simulink model "SolarPanelDigitalTwin_Auto"  (R2025b)
settings: Solver=ode23t  StartTime=0.0  StopTime=6300  MaxStep=4  RelTol=1e-3
libraries: ee_lib x117, fl_lib x9, nesl_utility x7, batteryecm_lib x1
settings Model: Creator=suraj  LastModifiedBy=suraj

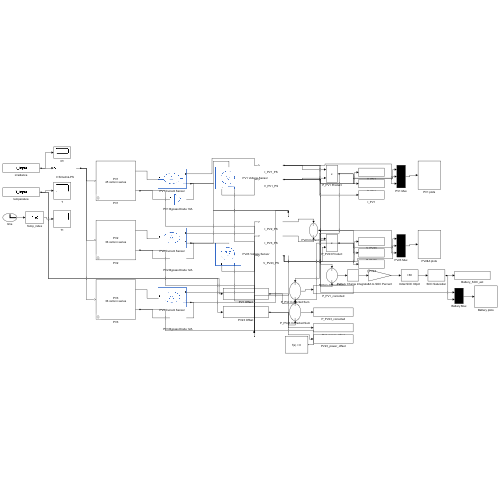
[thumbnail: Simulink's stored preview of the top-level diagram]
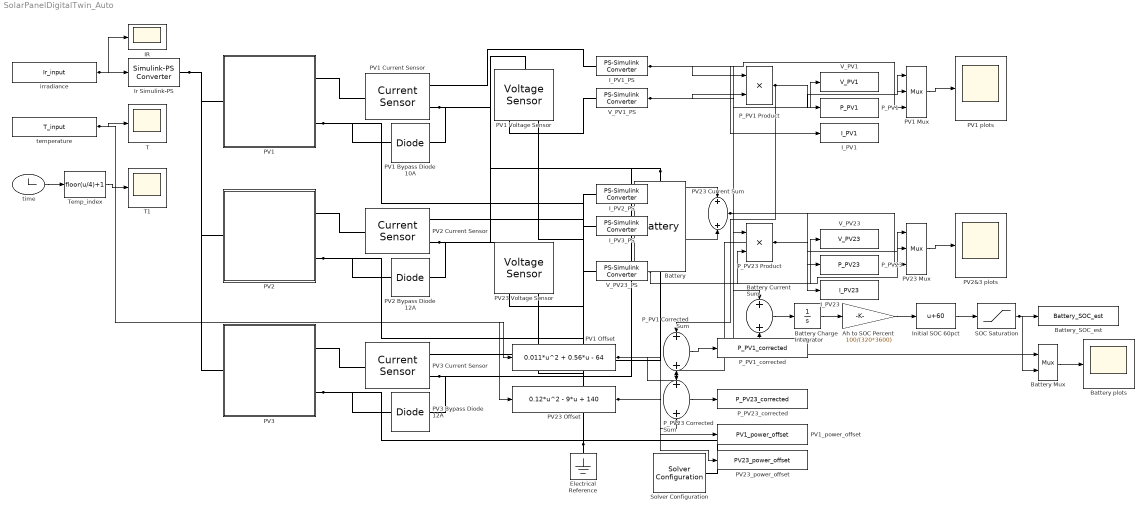
== system SolarPanelDigitalTwin_Auto ==
  Ah to SOC Percent : Gain  Gain=100/(320*3600)
  Battery : batteryecm_lib/Battery  Vnom=12 V  prm_dir=simscape.enum.battery.prm_dir.disabled  R1_dis=2 Ohm  R1_ch=2 Ohm  R1=0.05 Ohm  prm_AH=simscape.enum.battery.prm_AH.infinite  AH=320 A*hr  V1=11.5 V  AH1=25 A*hr  prm_R2=simscape.enum.battery.prm_R2.disabled  R2=2000 Ohm  Tmeas=298.15 K  charge_measurement_port=simscape.enum.battery.enable.no  prm_dyn=simscape.enum.battery.prm_dyn.off  Rp1=0.005 Ohm  tau1=30 s  Rp2=0.005 Ohm  tau2=30 s  Rp3=0.005 Ohm  tau3=30 s  Rp4=0.005 Ohm  tau4=30 s  Rp5=0.005 Ohm  tau5=30 s  prm_fade=simscape.enum.battery.prm_fade.disabled  N_fade=100  AH_fade=45 A*hr  R1_fade=2.02 Ohm  R1_ch_fade=2.02 Ohm  V1_fade=10.35 V  prm_age=simscape.enum.battery.prm_age.disabled  prm_age_OCV=simscape.enum.battery.prm_age_OCV.OCV  OCV_age=0.9  SOC_age=60  Tmeas_age=298.15 K  delta_time_age_vec=[0] d  temperature_age_vec=[273] K  OCV_scaling_age=2.2134e6  OCV_offset_age=1.632e6  temp_exp_age=0.515833569 V  t_exp_age=0.75  Vnom_T2=12 V  R1_T2=2.2 Ohm  R1_T2_dis=2.2 Ohm  R1_T2_ch=2.2 Ohm  V1_T2=11.4 V  R2_T2=2200 Ohm  Rp1_T2=0.005 Ohm  tau1_T2=30 s  Rp2_T2=0.005 Ohm  tau2_T2=30 s  Rp3_T2=0.005 Ohm  tau3_T2=30 s  Rp4_T2=0.005 Ohm  tau4_T2=30 s  Rp5_T2=0.005 Ohm  tau5_T2=30 s  Tmeas2=273.15 K  thermal_port=simscape.enum.thermaleffects.omit  thermal_mass=30000 J/K  i_specify=off  i_priority=None  i=0 A  i_nominal_specify=off  i_nominal_value=1  i_nominal_unit=A  v_specify=off  v_priority=None  v=0 V  v_nominal_specify=off  v_nominal_value=1  v_nominal_unit=V  charge_specify=off  charge_priority=High  charge=50 A*hr  charge_nominal_specify=off  charge_nominal_value=1  charge_nominal_unit=A*hr  num_cycles_specify=off  num_cycles_priority=High  num_cycles=0  num_cycles_nominal_specify=off  num_cycles_nominal_value=1  num_cycles_nominal_unit=1  temperature_specify=off  temperature_priority=High  temperature=298.15 K  temperature_nominal_specify=off  temperature_nominal_value=1  temperature_nominal_unit=K
  Battery Charge Integrator : Integrator
  Battery Current Sum : Sum
  Battery Mux : Mux  Inputs=2
  Battery plots : Scope
  Battery_SOC_est : ToWorkspace  VariableName=Battery_SOC_est  SampleTime=-1
  Electrical Reference : fl_lib/Electrical/Electrical Elements/Electrical Reference
  IR : Scope
  I_PV1 : ToWorkspace  VariableName=I_PV1  SampleTime=-1
  I_PV1_PS : nesl_utility/PS-Simulink Converter  PhysicalDomain=network_engine_domain  SubClassName=ps_output  LeftPortType=input  RightPortType=output  PseudoPeriodic=off  Frequencies=[]  VectorFormat=inherit  Unit=A  AffineConversion=off
  I_PV23 : ToWorkspace  VariableName=I_PV23  SampleTime=-1
  I_PV2_PS : nesl_utility/PS-Simulink Converter  PhysicalDomain=network_engine_domain  SubClassName=ps_output  LeftPortType=input  RightPortType=output  PseudoPeriodic=off  Frequencies=[]  VectorFormat=inherit  Unit=A  AffineConversion=off
  I_PV3_PS : nesl_utility/PS-Simulink Converter  PhysicalDomain=network_engine_domain  SubClassName=ps_output  LeftPortType=input  RightPortType=output  PseudoPeriodic=off  Frequencies=[]  VectorFormat=inherit  Unit=A  AffineConversion=off
  Initial SOC 60pct : Bias  Bias=60  SaturateOnIntegerOverflow=off
  Ir Simulink-PS : nesl_utility/Simulink-PS Converter  PhysicalDomain=network_engine_domain  SubClassName=ps_input  LeftPortType=input  RightPortType=output  PseudoPeriodic=off  Frequencies=[]  NoiseDistribution=none  NoiseParameters=[]  Unit=W/m^2  AffineConversion=off  FilteringAndDerivatives=provide  SimscapeFilterOrder=1  InputFilterTimeConstant=0.001  UdotUserProvided=0
  PV1 : Subsystem  mask{Isc=5.49, Voc=21.5, n=1.5, Rs=0, Ir0=1000, T=40}
      mask prompts: Isc "Short circuit current"; Voc "Open circuit voltage"; n "Quality factor, N"; Rs "Series resistance"; Ir0 "Reference irradiation"; T "Temperature"
      mask Display: disp('PV1\n45 cells in series')
  PV1 Bypass Diode 10A : fl_lib/Electrical/Electrical Elements/Diode  Vf=0.6 V  Ron=0.3 Ohm  Goff=1e-8 1/Ohm  i_specify=off  i_priority=None  i=0 A  i_nominal_specify=off  i_nominal_value=1  i_nominal_unit=A  v_specify=off  v_priority=None  v=0 V  v_nominal_specify=off  v_nominal_value=1  v_nominal_unit=V
  PV1 Current Sensor : fl_lib/Electrical/Electrical Sensors/Current Sensor
  PV1 Mux : Mux  Inputs=3
  PV1 Offset : Fcn  Expr=0.011*u^2 + 0.56*u - 64
  PV1 Voltage Sensor : fl_lib/Electrical/Electrical Sensors/Voltage Sensor
  PV1 plots : Scope
  PV1_power_offset : ToWorkspace  VariableName=PV1_power_offset  SampleTime=-1
  PV2 : Subsystem  mask{Isc=6.37, Voc=21.5, n=1.5, Rs=0, Ir0=1000, T=40}
      mask prompts: Isc "Short circuit current"; Voc "Open circuit voltage"; n "Quality factor, N"; Rs "Series resistance"; Ir0 "Reference irradiation"; T "Temperature"
      mask Display: disp('PV2\n36 cells in series')
  PV2 Bypass Diode 12A : fl_lib/Electrical/Electrical Elements/Diode  Vf=0.6 V  Ron=0.3 Ohm  Goff=1e-8 1/Ohm  i_specify=off  i_priority=None  i=0 A  i_nominal_specify=off  i_nominal_value=1  i_nominal_unit=A  v_specify=off  v_priority=None  v=0 V  v_nominal_specify=off  v_nominal_value=1  v_nominal_unit=V
  PV2 Current Sensor : fl_lib/Electrical/Electrical Sensors/Current Sensor
  PV2&3 plots : Scope
  PV23 Current Sum : Sum
  PV23 Mux : Mux  Inputs=3
  PV23 Offset : Fcn  Expr=0.12*u^2 - 9*u + 140
  PV23 Voltage Sensor : fl_lib/Electrical/Electrical Sensors/Voltage Sensor
  PV23_power_offset : ToWorkspace  VariableName=PV23_power_offset  SampleTime=-1
  PV3 : Subsystem  mask{Isc=6.37, Voc=21.5, n=1.5, Rs=0, Ir0=1000, T=40}
      mask prompts: Isc "Short circuit current"; Voc "Open circuit voltage"; n "Quality factor, N"; Rs "Series resistance"; Ir0 "Reference irradiation"; T "Temperature"
      mask Display: disp('PV3\n36 cells in series')
  PV3 Bypass Diode 12A : fl_lib/Electrical/Electrical Elements/Diode  Vf=0.6 V  Ron=0.3 Ohm  Goff=1e-8 1/Ohm  i_specify=off  i_priority=None  i=0 A  i_nominal_specify=off  i_nominal_value=1  i_nominal_unit=A  v_specify=off  v_priority=None  v=0 V  v_nominal_specify=off  v_nominal_value=1  v_nominal_unit=V
  PV3 Current Sensor : fl_lib/Electrical/Electrical Sensors/Current Sensor
  P_PV1 : ToWorkspace  VariableName=P_PV1  SampleTime=-1
  P_PV1 Corrected Sum : Sum
  P_PV1 Product : Product
  P_PV1_corrected : ToWorkspace  VariableName=P_PV1_corrected  SampleTime=-1
  P_PV23 : ToWorkspace  VariableName=P_PV23  SampleTime=-1
  P_PV23 Corrected Sum : Sum
  P_PV23 Product : Product
  P_PV23_corrected : ToWorkspace  VariableName=P_PV23_corrected  SampleTime=-1
  SOC Saturation : Saturate  UpperLimit=100  LowerLimit=0
  Solver Configuration : nesl_utility/Solver Configuration  PhysicalDomain=network_engine_domain  SubClassName=solver  LeftPortType=input  RightPortType=generic  Tones=[]  Harmonics=[]  SimulateNoise=off  Profile=off  UseLocalSampling=off  EnableSwitchedLinearOptims=on  FrequencyDomain=off  UseCCode=off  RelTol=0.001  AbsTol=0.001  MinStep=1e-09  ToWorkspace=off  RevertToSquareIcSolve=off  NumHomotopyIterations=100  PhasorMode=off  PhasorModeNumHarmonics=1  ConsistencySolver=NEWTON_XTOL_AFTER_FTOL  IndexReductionMethod=DerivativeReplacement  DoDC=on  ResidualTolerance=1e-09  ConsistencyTolSource=GLOBAL  ConsistencyAbsTol=0.001  ConsistencyRelTol=0.001  ConsistencyTolFactor=0.001  UseLocalSolver=off  LocalSolverChoice=NE_BACKWARD_EULER_ADVANCER  ResolveIndetEquations=on  FunctionEvalNumThread=1  LocalSolverSampleTime=4  DoFixedCost=off  MaxNonlinIter=3  MaxModeIter=2  ComputeImpulses=off  ImpulseIterations=2  LinearAlgebra=auto  LinearAlgebraNumThread=0  EquationFormulation=NE_TIME_EF  DelaysMemoryBudget=1024  AutomaticFiltering=on  FilteringTimeConstant=0.001  PartitionStorageMethod=AS_NEEDED  PartitionMemoryBudget=1024  PartitionMethod=ROBUST  MultibodyUseLocalSolver=off  MultibodyLocalSolverChoice=ODE1  MultibodyLocalSolverSampleTime=0.001
  T : Scope
  T1 : Scope
  Temp_index : Fcn  Expr=floor(u/4)+1
  V_PV1 : ToWorkspace  VariableName=V_PV1  SampleTime=-1
  V_PV1_PS : nesl_utility/PS-Simulink Converter  PhysicalDomain=network_engine_domain  SubClassName=ps_output  LeftPortType=input  RightPortType=output  PseudoPeriodic=off  Frequencies=[]  VectorFormat=inherit  Unit=V  AffineConversion=off
  V_PV23 : ToWorkspace  VariableName=V_PV23  SampleTime=-1
  V_PV23_PS : nesl_utility/PS-Simulink Converter  PhysicalDomain=network_engine_domain  SubClassName=ps_output  LeftPortType=input  RightPortType=output  PseudoPeriodic=off  Frequencies=[]  VectorFormat=inherit  Unit=V  AffineConversion=off
  irradiance : FromWorkspace  VariableName=Ir_input
  temperature : FromWorkspace  VariableName=T_input
  time : Clock
  wires:
  irradiance/1 -> Ir Simulink-PS/1, IR/1
  temperature/1 -> T/1, PV1 Offset/1, PV23 Offset/1
  time/1 -> Temp_index/1
  Temp_index/1 -> T1/1
  I_PV2_PS/1 -> PV23 Current Sum/1
  I_PV3_PS/1 -> PV23 Current Sum/2
  I_PV1_PS/1 -> P_PV1 Product/1, Battery Current Sum/1, I_PV1/1, PV1 Mux/3
  V_PV1_PS/1 -> P_PV1 Product/2, V_PV1/1, PV1 Mux/1, Battery Mux/1
  PV23 Current Sum/1 -> P_PV23 Product/1, Battery Current Sum/2, I_PV23/1, PV23 Mux/3
  V_PV23_PS/1 -> P_PV23 Product/2, V_PV23/1, PV23 Mux/1
  Battery Current Sum/1 -> Battery Charge Integrator/1
  Battery Charge Integrator/1 -> Ah to SOC Percent/1
  Ah to SOC Percent/1 -> Initial SOC 60pct/1
  Initial SOC 60pct/1 -> SOC Saturation/1
  P_PV1 Product/1 -> P_PV1/1, PV1 Mux/2, P_PV1 Corrected Sum/1
  P_PV23 Product/1 -> P_PV23/1, PV23 Mux/2, P_PV23 Corrected Sum/1
  SOC Saturation/1 -> Battery_SOC_est/1, Battery Mux/2
  PV1 Mux/1 -> PV1 plots/1
  PV23 Mux/1 -> PV2&3 plots/1
  Battery Mux/1 -> Battery plots/1
  PV1 Offset/1 -> P_PV1 Corrected Sum/2, PV1_power_offset/1
  PV23 Offset/1 -> P_PV23 Corrected Sum/2, PV23_power_offset/1
  P_PV1 Corrected Sum/1 -> P_PV1_corrected/1
  P_PV23 Corrected Sum/1 -> P_PV23_corrected/1
  connections:
  PV1/LConn1 -- Ir Simulink-PS/RConn1 -- PV2/LConn1 -- PV3/LConn1
  PV1/RConn1 -- PV1 Current Sensor/LConn1
  PV1 Current Sensor/RConn2 -- PV1 Voltage Sensor/LConn1 -- PV2 Current Sensor/RConn2 -- PV23 Voltage Sensor/LConn1 -- PV2 Bypass Diode 12A/RConn1 -- Battery/LConn1 -- PV3 Current Sensor/RConn2 -- PV3 Bypass Diode 12A/RConn1 -- PV1 Bypass Diode 10A/RConn1
  PV2/RConn1 -- PV2 Current Sensor/LConn1
  PV3/RConn1 -- PV3 Current Sensor/LConn1
  PV1/RConn2 -- PV1 Bypass Diode 10A/LConn1 -- PV2/RConn2 -- PV2 Bypass Diode 12A/LConn1 -- PV3/RConn2 -- PV3 Bypass Diode 12A/LConn1 -- Battery/RConn1 -- PV1 Voltage Sensor/RConn2 -- PV23 Voltage Sensor/RConn2 -- Electrical Reference/LConn1 -- Solver Configuration/RConn1
  PV1 Current Sensor/RConn1 -- I_PV1_PS/LConn1
  PV1 Voltage Sensor/RConn1 -- V_PV1_PS/LConn1
  PV2 Current Sensor/RConn1 -- I_PV2_PS/LConn1
  PV3 Current Sensor/RConn1 -- I_PV3_PS/LConn1
  PV23 Voltage Sensor/RConn1 -- V_PV23_PS/LConn1

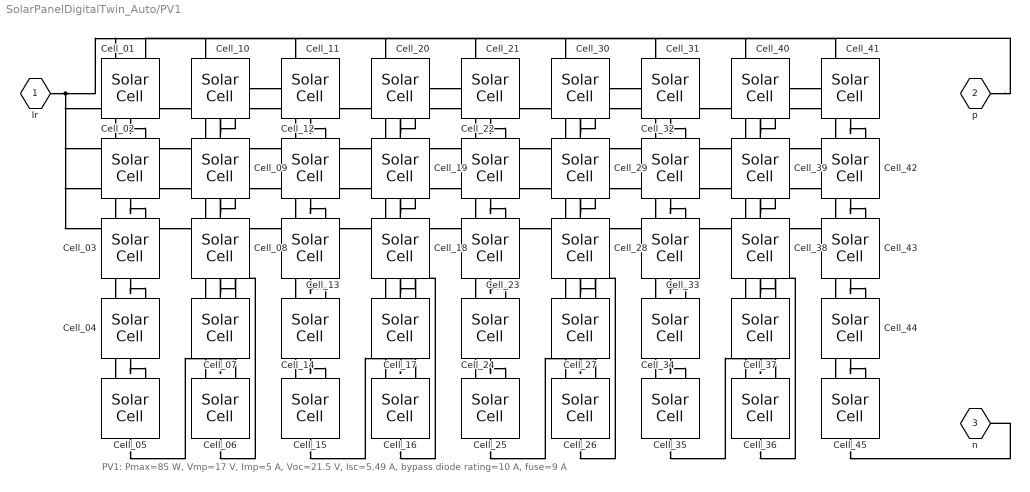
== system SolarPanelDigitalTwin_Auto/PV1 ==
  note: PV1: Pmax=85 W, Vmp=17 V, Imp=5 A, Voc=21.5 V, Isc=5.49 A, bypass diode rating=10 A, fuse=9 A
  Cell_01 : ee_lib/Sources/Solar Cell  prm=ee.enum.sources.solar_cell_prm.datasheet  Isc=Isc A  Voc=Voc/45 V  Is=1e-6 A  Is2=0 A  Iph=7.34 A  Ir0=Ir0 W/m^2  ec=n  N2=2  Rs=Rs/45 Ohm  Rp=inf Ohm  N_series=1  N_parallel=1  TIPH1=0 1/K  EG=1.11 eV  TXIS1=3  TXIS2=3  TRS1=0  TRP1=0  Tmeas=T degC  TFIXED=T degC  thermal_mass=100 J/K  initial_temperature=25 degC
  Cell_02 : ee_lib/Sources/Solar Cell  prm=ee.enum.sources.solar_cell_prm.datasheet  Isc=Isc A  Voc=Voc/45 V  Is=1e-6 A  Is2=0 A  Iph=7.34 A  Ir0=Ir0 W/m^2  ec=n  N2=2  Rs=Rs/45 Ohm  Rp=inf Ohm  N_series=1  N_parallel=1  TIPH1=0 1/K  EG=1.11 eV  TXIS1=3  TXIS2=3  TRS1=0  TRP1=0  Tmeas=T degC  TFIXED=T degC  thermal_mass=100 J/K  initial_temperature=25 degC
  Cell_03 : ee_lib/Sources/Solar Cell  prm=ee.enum.sources.solar_cell_prm.datasheet  Isc=Isc A  Voc=Voc/45 V  Is=1e-6 A  Is2=0 A  Iph=7.34 A  Ir0=Ir0 W/m^2  ec=n  N2=2  Rs=Rs/45 Ohm  Rp=inf Ohm  N_series=1  N_parallel=1  TIPH1=0 1/K  EG=1.11 eV  TXIS1=3  TXIS2=3  TRS1=0  TRP1=0  Tmeas=T degC  TFIXED=T degC  thermal_mass=100 J/K  initial_temperature=25 degC
  Cell_04 : ee_lib/Sources/Solar Cell  prm=ee.enum.sources.solar_cell_prm.datasheet  Isc=Isc A  Voc=Voc/45 V  Is=1e-6 A  Is2=0 A  Iph=7.34 A  Ir0=Ir0 W/m^2  ec=n  N2=2  Rs=Rs/45 Ohm  Rp=inf Ohm  N_series=1  N_parallel=1  TIPH1=0 1/K  EG=1.11 eV  TXIS1=3  TXIS2=3  TRS1=0  TRP1=0  Tmeas=T degC  TFIXED=T degC  thermal_mass=100 J/K  initial_temperature=25 degC
  Cell_05 : ee_lib/Sources/Solar Cell  prm=ee.enum.sources.solar_cell_prm.datasheet  Isc=Isc A  Voc=Voc/45 V  Is=1e-6 A  Is2=0 A  Iph=7.34 A  Ir0=Ir0 W/m^2  ec=n  N2=2  Rs=Rs/45 Ohm  Rp=inf Ohm  N_series=1  N_parallel=1  TIPH1=0 1/K  EG=1.11 eV  TXIS1=3  TXIS2=3  TRS1=0  TRP1=0  Tmeas=T degC  TFIXED=T degC  thermal_mass=100 J/K  initial_temperature=25 degC
  Cell_06 : ee_lib/Sources/Solar Cell  prm=ee.enum.sources.solar_cell_prm.datasheet  Isc=Isc A  Voc=Voc/45 V  Is=1e-6 A  Is2=0 A  Iph=7.34 A  Ir0=Ir0 W/m^2  ec=n  N2=2  Rs=Rs/45 Ohm  Rp=inf Ohm  N_series=1  N_parallel=1  TIPH1=0 1/K  EG=1.11 eV  TXIS1=3  TXIS2=3  TRS1=0  TRP1=0  Tmeas=T degC  TFIXED=T degC  thermal_mass=100 J/K  initial_temperature=25 degC
  Cell_07 : ee_lib/Sources/Solar Cell  prm=ee.enum.sources.solar_cell_prm.datasheet  Isc=Isc A  Voc=Voc/45 V  Is=1e-6 A  Is2=0 A  Iph=7.34 A  Ir0=Ir0 W/m^2  ec=n  N2=2  Rs=Rs/45 Ohm  Rp=inf Ohm  N_series=1  N_parallel=1  TIPH1=0 1/K  EG=1.11 eV  TXIS1=3  TXIS2=3  TRS1=0  TRP1=0  Tmeas=T degC  TFIXED=T degC  thermal_mass=100 J/K  initial_temperature=25 degC
  Cell_08 : ee_lib/Sources/Solar Cell  prm=ee.enum.sources.solar_cell_prm.datasheet  Isc=Isc A  Voc=Voc/45 V  Is=1e-6 A  Is2=0 A  Iph=7.34 A  Ir0=Ir0 W/m^2  ec=n  N2=2  Rs=Rs/45 Ohm  Rp=inf Ohm  N_series=1  N_parallel=1  TIPH1=0 1/K  EG=1.11 eV  TXIS1=3  TXIS2=3  TRS1=0  TRP1=0  Tmeas=T degC  TFIXED=T degC  thermal_mass=100 J/K  initial_temperature=25 degC
  Cell_09 : ee_lib/Sources/Solar Cell  prm=ee.enum.sources.solar_cell_prm.datasheet  Isc=Isc A  Voc=Voc/45 V  Is=1e-6 A  Is2=0 A  Iph=7.34 A  Ir0=Ir0 W/m^2  ec=n  N2=2  Rs=Rs/45 Ohm  Rp=inf Ohm  N_series=1  N_parallel=1  TIPH1=0 1/K  EG=1.11 eV  TXIS1=3  TXIS2=3  TRS1=0  TRP1=0  Tmeas=T degC  TFIXED=T degC  thermal_mass=100 J/K  initial_temperature=25 degC
  Cell_{10..45} (36 alike) : ee_lib/Sources/Solar Cell  prm=ee.enum.sources.solar_cell_prm.datasheet  Isc=Isc A  Voc=Voc/45 V  Is=1e-6 A  Is2=0 A  Iph=7.34 A  Ir0=Ir0 W/m^2  ec=n  N2=2  Rs=Rs/45 Ohm  Rp=inf Ohm  N_series=1  N_parallel=1  TIPH1=0 1/K  EG=1.11 eV  TXIS1=3  TXIS2=3  TRS1=0  TRP1=0  Tmeas=T degC  TFIXED=T degC  thermal_mass=100 J/K  initial_temperature=25 degC
  Ir : PMIOPort  Side=Left
  p : PMIOPort  Port=2  Side=Right
  n : PMIOPort  Port=3  Side=Right
  wires:
  ? -> ?
  connections:
  Cell_01/LConn1 -- Ir/RConn1 -- Cell_02/LConn1 -- Cell_03/LConn1 -- Cell_04/LConn1 -- Cell_05/LConn1 -- Cell_06/LConn1 -- Cell_07/LConn1 -- Cell_08/LConn1 -- Cell_09/LConn1 -- Cell_10/LConn1 -- Cell_11/LConn1 -- Cell_12/LConn1 -- Cell_13/LConn1 -- Cell_14/LConn1 -- Cell_15/LConn1 -- Cell_16/LConn1 -- Cell_17/LConn1 -- Cell_18/LConn1 -- Cell_19/LConn1 -- Cell_20/LConn1 -- Cell_21/LConn1 -- Cell_22/LConn1 -- Cell_23/LConn1 -- Cell_24/LConn1 -- Cell_25/LConn1 -- Cell_26/LConn1 -- Cell_27/LConn1 -- Cell_28/LConn1 -- Cell_29/LConn1 -- Cell_30/LConn1 -- Cell_31/LConn1 -- Cell_32/LConn1 -- Cell_33/LConn1 -- Cell_34/LConn1 -- Cell_35/LConn1 -- Cell_36/LConn1 -- Cell_37/LConn1 -- Cell_38/LConn1 -- Cell_39/LConn1 -- Cell_40/LConn1 -- Cell_41/LConn1 -- Cell_42/LConn1 -- Cell_43/LConn1 -- Cell_44/LConn1 -- Cell_45/LConn1
  Cell_01/RConn1 -- Cell_02/LConn2
  Cell_02/RConn1 -- Cell_03/LConn2
  Cell_03/RConn1 -- Cell_04/LConn2
  Cell_04/RConn1 -- Cell_05/LConn2
  Cell_05/RConn1 -- Cell_06/LConn2
  Cell_06/RConn1 -- Cell_07/LConn2
  Cell_07/RConn1 -- Cell_08/LConn2
  Cell_08/RConn1 -- Cell_09/LConn2
  Cell_09/RConn1 -- Cell_10/LConn2
  Cell_10/RConn1 -- Cell_11/LConn2
  Cell_11/RConn1 -- Cell_12/LConn2
  Cell_12/RConn1 -- Cell_13/LConn2
  Cell_13/RConn1 -- Cell_14/LConn2
  Cell_14/RConn1 -- Cell_15/LConn2
  Cell_15/RConn1 -- Cell_16/LConn2
  Cell_16/RConn1 -- Cell_17/LConn2
  Cell_17/RConn1 -- Cell_18/LConn2
  Cell_18/RConn1 -- Cell_19/LConn2
  Cell_19/RConn1 -- Cell_20/LConn2
  Cell_20/RConn1 -- Cell_21/LConn2
  Cell_21/RConn1 -- Cell_22/LConn2
  Cell_22/RConn1 -- Cell_23/LConn2
  Cell_23/RConn1 -- Cell_24/LConn2
  Cell_24/RConn1 -- Cell_25/LConn2
  Cell_25/RConn1 -- Cell_26/LConn2
  Cell_26/RConn1 -- Cell_27/LConn2
  Cell_27/RConn1 -- Cell_28/LConn2
  Cell_28/RConn1 -- Cell_29/LConn2
  Cell_29/RConn1 -- Cell_30/LConn2
  Cell_30/RConn1 -- Cell_31/LConn2
  Cell_31/RConn1 -- Cell_32/LConn2
  Cell_32/RConn1 -- Cell_33/LConn2
  Cell_33/RConn1 -- Cell_34/LConn2
  Cell_34/RConn1 -- Cell_35/LConn2
  Cell_35/RConn1 -- Cell_36/LConn2
  Cell_36/RConn1 -- Cell_37/LConn2
  Cell_37/RConn1 -- Cell_38/LConn2
  Cell_38/RConn1 -- Cell_39/LConn2
  Cell_39/RConn1 -- Cell_40/LConn2
  Cell_40/RConn1 -- Cell_41/LConn2
  Cell_41/RConn1 -- Cell_42/LConn2
  Cell_42/RConn1 -- Cell_43/LConn2
  Cell_43/RConn1 -- Cell_44/LConn2
  Cell_44/RConn1 -- Cell_45/LConn2
  p/RConn1 -- Cell_01/LConn2
  Cell_45/RConn1 -- n/RConn1

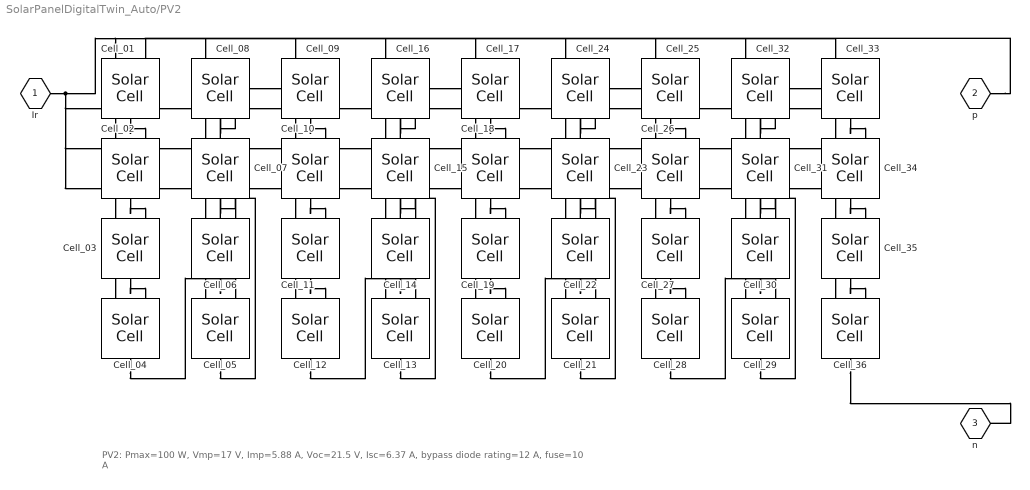
== system SolarPanelDigitalTwin_Auto/PV2 ==
  note: PV2: Pmax=100 W, Vmp=17 V, Imp=5.88 A, Voc=21.5 V, Isc=6.37 A, bypass diode rating=12 A, fuse=10 A
  Cell_01 : ee_lib/Sources/Solar Cell  prm=ee.enum.sources.solar_cell_prm.datasheet  Isc=Isc A  Voc=Voc/36 V  Is=1e-6 A  Is2=0 A  Iph=7.34 A  Ir0=Ir0 W/m^2  ec=n  N2=2  Rs=Rs/36 Ohm  Rp=inf Ohm  N_series=1  N_parallel=1  TIPH1=0 1/K  EG=1.11 eV  TXIS1=3  TXIS2=3  TRS1=0  TRP1=0  Tmeas=T degC  TFIXED=T degC  thermal_mass=100 J/K  initial_temperature=25 degC
  Cell_02 : ee_lib/Sources/Solar Cell  prm=ee.enum.sources.solar_cell_prm.datasheet  Isc=Isc A  Voc=Voc/36 V  Is=1e-6 A  Is2=0 A  Iph=7.34 A  Ir0=Ir0 W/m^2  ec=n  N2=2  Rs=Rs/36 Ohm  Rp=inf Ohm  N_series=1  N_parallel=1  TIPH1=0 1/K  EG=1.11 eV  TXIS1=3  TXIS2=3  TRS1=0  TRP1=0  Tmeas=T degC  TFIXED=T degC  thermal_mass=100 J/K  initial_temperature=25 degC
  Cell_03 : ee_lib/Sources/Solar Cell  prm=ee.enum.sources.solar_cell_prm.datasheet  Isc=Isc A  Voc=Voc/36 V  Is=1e-6 A  Is2=0 A  Iph=7.34 A  Ir0=Ir0 W/m^2  ec=n  N2=2  Rs=Rs/36 Ohm  Rp=inf Ohm  N_series=1  N_parallel=1  TIPH1=0 1/K  EG=1.11 eV  TXIS1=3  TXIS2=3  TRS1=0  TRP1=0  Tmeas=T degC  TFIXED=T degC  thermal_mass=100 J/K  initial_temperature=25 degC
  Cell_04 : ee_lib/Sources/Solar Cell  prm=ee.enum.sources.solar_cell_prm.datasheet  Isc=Isc A  Voc=Voc/36 V  Is=1e-6 A  Is2=0 A  Iph=7.34 A  Ir0=Ir0 W/m^2  ec=n  N2=2  Rs=Rs/36 Ohm  Rp=inf Ohm  N_series=1  N_parallel=1  TIPH1=0 1/K  EG=1.11 eV  TXIS1=3  TXIS2=3  TRS1=0  TRP1=0  Tmeas=T degC  TFIXED=T degC  thermal_mass=100 J/K  initial_temperature=25 degC
  Cell_05 : ee_lib/Sources/Solar Cell  prm=ee.enum.sources.solar_cell_prm.datasheet  Isc=Isc A  Voc=Voc/36 V  Is=1e-6 A  Is2=0 A  Iph=7.34 A  Ir0=Ir0 W/m^2  ec=n  N2=2  Rs=Rs/36 Ohm  Rp=inf Ohm  N_series=1  N_parallel=1  TIPH1=0 1/K  EG=1.11 eV  TXIS1=3  TXIS2=3  TRS1=0  TRP1=0  Tmeas=T degC  TFIXED=T degC  thermal_mass=100 J/K  initial_temperature=25 degC
  Cell_06 : ee_lib/Sources/Solar Cell  prm=ee.enum.sources.solar_cell_prm.datasheet  Isc=Isc A  Voc=Voc/36 V  Is=1e-6 A  Is2=0 A  Iph=7.34 A  Ir0=Ir0 W/m^2  ec=n  N2=2  Rs=Rs/36 Ohm  Rp=inf Ohm  N_series=1  N_parallel=1  TIPH1=0 1/K  EG=1.11 eV  TXIS1=3  TXIS2=3  TRS1=0  TRP1=0  Tmeas=T degC  TFIXED=T degC  thermal_mass=100 J/K  initial_temperature=25 degC
  Cell_07 : ee_lib/Sources/Solar Cell  prm=ee.enum.sources.solar_cell_prm.datasheet  Isc=Isc A  Voc=Voc/36 V  Is=1e-6 A  Is2=0 A  Iph=7.34 A  Ir0=Ir0 W/m^2  ec=n  N2=2  Rs=Rs/36 Ohm  Rp=inf Ohm  N_series=1  N_parallel=1  TIPH1=0 1/K  EG=1.11 eV  TXIS1=3  TXIS2=3  TRS1=0  TRP1=0  Tmeas=T degC  TFIXED=T degC  thermal_mass=100 J/K  initial_temperature=25 degC
  Cell_08 : ee_lib/Sources/Solar Cell  prm=ee.enum.sources.solar_cell_prm.datasheet  Isc=Isc A  Voc=Voc/36 V  Is=1e-6 A  Is2=0 A  Iph=7.34 A  Ir0=Ir0 W/m^2  ec=n  N2=2  Rs=Rs/36 Ohm  Rp=inf Ohm  N_series=1  N_parallel=1  TIPH1=0 1/K  EG=1.11 eV  TXIS1=3  TXIS2=3  TRS1=0  TRP1=0  Tmeas=T degC  TFIXED=T degC  thermal_mass=100 J/K  initial_temperature=25 degC
  Cell_09 : ee_lib/Sources/Solar Cell  prm=ee.enum.sources.solar_cell_prm.datasheet  Isc=Isc A  Voc=Voc/36 V  Is=1e-6 A  Is2=0 A  Iph=7.34 A  Ir0=Ir0 W/m^2  ec=n  N2=2  Rs=Rs/36 Ohm  Rp=inf Ohm  N_series=1  N_parallel=1  TIPH1=0 1/K  EG=1.11 eV  TXIS1=3  TXIS2=3  TRS1=0  TRP1=0  Tmeas=T degC  TFIXED=T degC  thermal_mass=100 J/K  initial_temperature=25 degC
  Cell_{10..36} (27 alike) : ee_lib/Sources/Solar Cell  prm=ee.enum.sources.solar_cell_prm.datasheet  Isc=Isc A  Voc=Voc/36 V  Is=1e-6 A  Is2=0 A  Iph=7.34 A  Ir0=Ir0 W/m^2  ec=n  N2=2  Rs=Rs/36 Ohm  Rp=inf Ohm  N_series=1  N_parallel=1  TIPH1=0 1/K  EG=1.11 eV  TXIS1=3  TXIS2=3  TRS1=0  TRP1=0  Tmeas=T degC  TFIXED=T degC  thermal_mass=100 J/K  initial_temperature=25 degC
  Ir : PMIOPort  Side=Left
  p : PMIOPort  Port=2  Side=Right
  n : PMIOPort  Port=3  Side=Right
  wires:
  ? -> ?
  connections:
  Cell_01/LConn1 -- Ir/RConn1 -- Cell_02/LConn1 -- Cell_03/LConn1 -- Cell_04/LConn1 -- Cell_05/LConn1 -- Cell_06/LConn1 -- Cell_07/LConn1 -- Cell_08/LConn1 -- Cell_09/LConn1 -- Cell_10/LConn1 -- Cell_11/LConn1 -- Cell_12/LConn1 -- Cell_13/LConn1 -- Cell_14/LConn1 -- Cell_15/LConn1 -- Cell_16/LConn1 -- Cell_17/LConn1 -- Cell_18/LConn1 -- Cell_19/LConn1 -- Cell_20/LConn1 -- Cell_21/LConn1 -- Cell_22/LConn1 -- Cell_23/LConn1 -- Cell_24/LConn1 -- Cell_25/LConn1 -- Cell_26/LConn1 -- Cell_27/LConn1 -- Cell_28/LConn1 -- Cell_29/LConn1 -- Cell_30/LConn1 -- Cell_31/LConn1 -- Cell_32/LConn1 -- Cell_33/LConn1 -- Cell_34/LConn1 -- Cell_35/LConn1 -- Cell_36/LConn1
  Cell_01/RConn1 -- Cell_02/LConn2
  Cell_02/RConn1 -- Cell_03/LConn2
  Cell_03/RConn1 -- Cell_04/LConn2
  Cell_04/RConn1 -- Cell_05/LConn2
  Cell_05/RConn1 -- Cell_06/LConn2
  Cell_06/RConn1 -- Cell_07/LConn2
  Cell_07/RConn1 -- Cell_08/LConn2
  Cell_08/RConn1 -- Cell_09/LConn2
  Cell_09/RConn1 -- Cell_10/LConn2
  Cell_10/RConn1 -- Cell_11/LConn2
  Cell_11/RConn1 -- Cell_12/LConn2
  Cell_12/RConn1 -- Cell_13/LConn2
  Cell_13/RConn1 -- Cell_14/LConn2
  Cell_14/RConn1 -- Cell_15/LConn2
  Cell_15/RConn1 -- Cell_16/LConn2
  Cell_16/RConn1 -- Cell_17/LConn2
  Cell_17/RConn1 -- Cell_18/LConn2
  Cell_18/RConn1 -- Cell_19/LConn2
  Cell_19/RConn1 -- Cell_20/LConn2
  Cell_20/RConn1 -- Cell_21/LConn2
  Cell_21/RConn1 -- Cell_22/LConn2
  Cell_22/RConn1 -- Cell_23/LConn2
  Cell_23/RConn1 -- Cell_24/LConn2
  Cell_24/RConn1 -- Cell_25/LConn2
  Cell_25/RConn1 -- Cell_26/LConn2
  Cell_26/RConn1 -- Cell_27/LConn2
  Cell_27/RConn1 -- Cell_28/LConn2
  Cell_28/RConn1 -- Cell_29/LConn2
  Cell_29/RConn1 -- Cell_30/LConn2
  Cell_30/RConn1 -- Cell_31/LConn2
  Cell_31/RConn1 -- Cell_32/LConn2
  Cell_32/RConn1 -- Cell_33/LConn2
  Cell_33/RConn1 -- Cell_34/LConn2
  Cell_34/RConn1 -- Cell_35/LConn2
  Cell_35/RConn1 -- Cell_36/LConn2
  p/RConn1 -- Cell_01/LConn2
  Cell_36/RConn1 -- n/RConn1

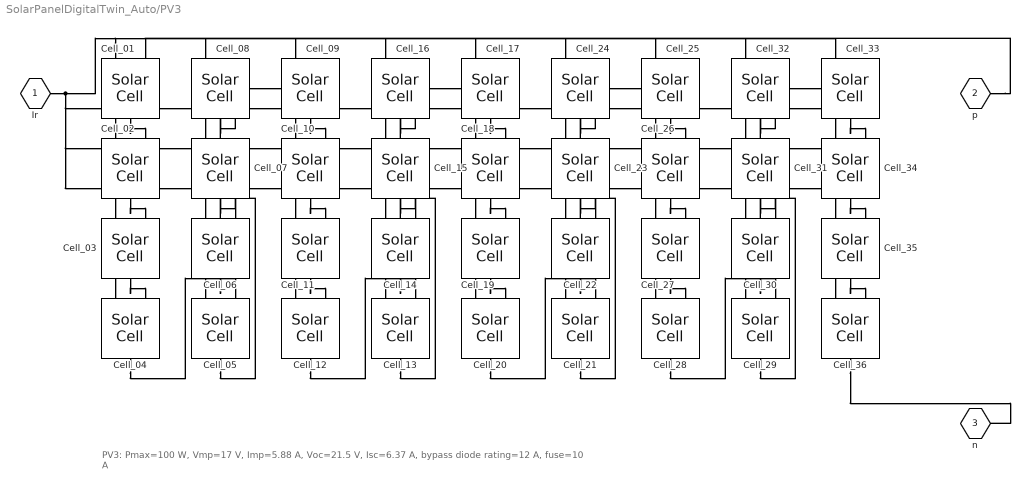
== system SolarPanelDigitalTwin_Auto/PV3 ==
  note: PV3: Pmax=100 W, Vmp=17 V, Imp=5.88 A, Voc=21.5 V, Isc=6.37 A, bypass diode rating=12 A, fuse=10 A
  Cell_01 : ee_lib/Sources/Solar Cell  prm=ee.enum.sources.solar_cell_prm.datasheet  Isc=Isc A  Voc=Voc/36 V  Is=1e-6 A  Is2=0 A  Iph=7.34 A  Ir0=Ir0 W/m^2  ec=n  N2=2  Rs=Rs/36 Ohm  Rp=inf Ohm  N_series=1  N_parallel=1  TIPH1=0 1/K  EG=1.11 eV  TXIS1=3  TXIS2=3  TRS1=0  TRP1=0  Tmeas=T degC  TFIXED=T degC  thermal_mass=100 J/K  initial_temperature=25 degC
  Cell_02 : ee_lib/Sources/Solar Cell  prm=ee.enum.sources.solar_cell_prm.datasheet  Isc=Isc A  Voc=Voc/36 V  Is=1e-6 A  Is2=0 A  Iph=7.34 A  Ir0=Ir0 W/m^2  ec=n  N2=2  Rs=Rs/36 Ohm  Rp=inf Ohm  N_series=1  N_parallel=1  TIPH1=0 1/K  EG=1.11 eV  TXIS1=3  TXIS2=3  TRS1=0  TRP1=0  Tmeas=T degC  TFIXED=T degC  thermal_mass=100 J/K  initial_temperature=25 degC
  Cell_03 : ee_lib/Sources/Solar Cell  prm=ee.enum.sources.solar_cell_prm.datasheet  Isc=Isc A  Voc=Voc/36 V  Is=1e-6 A  Is2=0 A  Iph=7.34 A  Ir0=Ir0 W/m^2  ec=n  N2=2  Rs=Rs/36 Ohm  Rp=inf Ohm  N_series=1  N_parallel=1  TIPH1=0 1/K  EG=1.11 eV  TXIS1=3  TXIS2=3  TRS1=0  TRP1=0  Tmeas=T degC  TFIXED=T degC  thermal_mass=100 J/K  initial_temperature=25 degC
  Cell_04 : ee_lib/Sources/Solar Cell  prm=ee.enum.sources.solar_cell_prm.datasheet  Isc=Isc A  Voc=Voc/36 V  Is=1e-6 A  Is2=0 A  Iph=7.34 A  Ir0=Ir0 W/m^2  ec=n  N2=2  Rs=Rs/36 Ohm  Rp=inf Ohm  N_series=1  N_parallel=1  TIPH1=0 1/K  EG=1.11 eV  TXIS1=3  TXIS2=3  TRS1=0  TRP1=0  Tmeas=T degC  TFIXED=T degC  thermal_mass=100 J/K  initial_temperature=25 degC
  Cell_05 : ee_lib/Sources/Solar Cell  prm=ee.enum.sources.solar_cell_prm.datasheet  Isc=Isc A  Voc=Voc/36 V  Is=1e-6 A  Is2=0 A  Iph=7.34 A  Ir0=Ir0 W/m^2  ec=n  N2=2  Rs=Rs/36 Ohm  Rp=inf Ohm  N_series=1  N_parallel=1  TIPH1=0 1/K  EG=1.11 eV  TXIS1=3  TXIS2=3  TRS1=0  TRP1=0  Tmeas=T degC  TFIXED=T degC  thermal_mass=100 J/K  initial_temperature=25 degC
  Cell_06 : ee_lib/Sources/Solar Cell  prm=ee.enum.sources.solar_cell_prm.datasheet  Isc=Isc A  Voc=Voc/36 V  Is=1e-6 A  Is2=0 A  Iph=7.34 A  Ir0=Ir0 W/m^2  ec=n  N2=2  Rs=Rs/36 Ohm  Rp=inf Ohm  N_series=1  N_parallel=1  TIPH1=0 1/K  EG=1.11 eV  TXIS1=3  TXIS2=3  TRS1=0  TRP1=0  Tmeas=T degC  TFIXED=T degC  thermal_mass=100 J/K  initial_temperature=25 degC
  Cell_07 : ee_lib/Sources/Solar Cell  prm=ee.enum.sources.solar_cell_prm.datasheet  Isc=Isc A  Voc=Voc/36 V  Is=1e-6 A  Is2=0 A  Iph=7.34 A  Ir0=Ir0 W/m^2  ec=n  N2=2  Rs=Rs/36 Ohm  Rp=inf Ohm  N_series=1  N_parallel=1  TIPH1=0 1/K  EG=1.11 eV  TXIS1=3  TXIS2=3  TRS1=0  TRP1=0  Tmeas=T degC  TFIXED=T degC  thermal_mass=100 J/K  initial_temperature=25 degC
  Cell_08 : ee_lib/Sources/Solar Cell  prm=ee.enum.sources.solar_cell_prm.datasheet  Isc=Isc A  Voc=Voc/36 V  Is=1e-6 A  Is2=0 A  Iph=7.34 A  Ir0=Ir0 W/m^2  ec=n  N2=2  Rs=Rs/36 Ohm  Rp=inf Ohm  N_series=1  N_parallel=1  TIPH1=0 1/K  EG=1.11 eV  TXIS1=3  TXIS2=3  TRS1=0  TRP1=0  Tmeas=T degC  TFIXED=T degC  thermal_mass=100 J/K  initial_temperature=25 degC
  Cell_09 : ee_lib/Sources/Solar Cell  prm=ee.enum.sources.solar_cell_prm.datasheet  Isc=Isc A  Voc=Voc/36 V  Is=1e-6 A  Is2=0 A  Iph=7.34 A  Ir0=Ir0 W/m^2  ec=n  N2=2  Rs=Rs/36 Ohm  Rp=inf Ohm  N_series=1  N_parallel=1  TIPH1=0 1/K  EG=1.11 eV  TXIS1=3  TXIS2=3  TRS1=0  TRP1=0  Tmeas=T degC  TFIXED=T degC  thermal_mass=100 J/K  initial_temperature=25 degC
  Cell_{10..36} (27 alike) : ee_lib/Sources/Solar Cell  prm=ee.enum.sources.solar_cell_prm.datasheet  Isc=Isc A  Voc=Voc/36 V  Is=1e-6 A  Is2=0 A  Iph=7.34 A  Ir0=Ir0 W/m^2  ec=n  N2=2  Rs=Rs/36 Ohm  Rp=inf Ohm  N_series=1  N_parallel=1  TIPH1=0 1/K  EG=1.11 eV  TXIS1=3  TXIS2=3  TRS1=0  TRP1=0  Tmeas=T degC  TFIXED=T degC  thermal_mass=100 J/K  initial_temperature=25 degC
  Ir : PMIOPort  Side=Left
  p : PMIOPort  Port=2  Side=Right
  n : PMIOPort  Port=3  Side=Right
  wires:
  ? -> ?
  connections:
  Cell_01/LConn1 -- Ir/RConn1 -- Cell_02/LConn1 -- Cell_03/LConn1 -- Cell_04/LConn1 -- Cell_05/LConn1 -- Cell_06/LConn1 -- Cell_07/LConn1 -- Cell_08/LConn1 -- Cell_09/LConn1 -- Cell_10/LConn1 -- Cell_11/LConn1 -- Cell_12/LConn1 -- Cell_13/LConn1 -- Cell_14/LConn1 -- Cell_15/LConn1 -- Cell_16/LConn1 -- Cell_17/LConn1 -- Cell_18/LConn1 -- Cell_19/LConn1 -- Cell_20/LConn1 -- Cell_21/LConn1 -- Cell_22/LConn1 -- Cell_23/LConn1 -- Cell_24/LConn1 -- Cell_25/LConn1 -- Cell_26/LConn1 -- Cell_27/LConn1 -- Cell_28/LConn1 -- Cell_29/LConn1 -- Cell_30/LConn1 -- Cell_31/LConn1 -- Cell_32/LConn1 -- Cell_33/LConn1 -- Cell_34/LConn1 -- Cell_35/LConn1 -- Cell_36/LConn1
  Cell_01/RConn1 -- Cell_02/LConn2
  Cell_02/RConn1 -- Cell_03/LConn2
  Cell_03/RConn1 -- Cell_04/LConn2
  Cell_04/RConn1 -- Cell_05/LConn2
  Cell_05/RConn1 -- Cell_06/LConn2
  Cell_06/RConn1 -- Cell_07/LConn2
  Cell_07/RConn1 -- Cell_08/LConn2
  Cell_08/RConn1 -- Cell_09/LConn2
  Cell_09/RConn1 -- Cell_10/LConn2
  Cell_10/RConn1 -- Cell_11/LConn2
  Cell_11/RConn1 -- Cell_12/LConn2
  Cell_12/RConn1 -- Cell_13/LConn2
  Cell_13/RConn1 -- Cell_14/LConn2
  Cell_14/RConn1 -- Cell_15/LConn2
  Cell_15/RConn1 -- Cell_16/LConn2
  Cell_16/RConn1 -- Cell_17/LConn2
  Cell_17/RConn1 -- Cell_18/LConn2
  Cell_18/RConn1 -- Cell_19/LConn2
  Cell_19/RConn1 -- Cell_20/LConn2
  Cell_20/RConn1 -- Cell_21/LConn2
  Cell_21/RConn1 -- Cell_22/LConn2
  Cell_22/RConn1 -- Cell_23/LConn2
  Cell_23/RConn1 -- Cell_24/LConn2
  Cell_24/RConn1 -- Cell_25/LConn2
  Cell_25/RConn1 -- Cell_26/LConn2
  Cell_26/RConn1 -- Cell_27/LConn2
  Cell_27/RConn1 -- Cell_28/LConn2
  Cell_28/RConn1 -- Cell_29/LConn2
  Cell_29/RConn1 -- Cell_30/LConn2
  Cell_30/RConn1 -- Cell_31/LConn2
  Cell_31/RConn1 -- Cell_32/LConn2
  Cell_32/RConn1 -- Cell_33/LConn2
  Cell_33/RConn1 -- Cell_34/LConn2
  Cell_34/RConn1 -- Cell_35/LConn2
  Cell_35/RConn1 -- Cell_36/LConn2
  p/RConn1 -- Cell_01/LConn2
  Cell_36/RConn1 -- n/RConn1
